simulink model "Loops6"  (Simulink 8.7)
settings: Solver=ode45  StartTime=0.0  StopTime=10.0  RelTol=1e-3
settings Model: Creator=scaife  LastModifiedBy=bourbouh  ExtModeAutoUpdateStatusClock=off
settings DataIOCC: SignalLoggingSaveFormat=ModelDataLogs  SignalLoggingName=sigsOut
settings OptimizationCC: InitFltsAndDblsToZero=on
settings DebuggingCC: SaveWithParameterizedLinksMsg=none  SignalResolutionControl=TryResolveAllWithWarning  MultiTaskDSMMsg=warning  MultiTaskCondExecSysMsg=none
settings HardwareCC: TargetUnknown=on
settings SFSimCC: SimParseCustomCode=off
settings GRTTargetCC: TargetFcnLib=ansi_tfl_tmw.mat  ModelReferenceCompliant=off  GeneratePreprocessorConditionals=Use local settings  CombineOutputUpdateFcns=off  MatFileLogging=off  GRTInterface=on

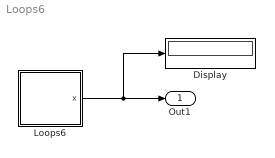
== system Loops6 ==
  Display : Display
  Loops6 : Stateflow chart  TreatAsAtomicUnit=on
  Out1 : Outport
  wires:
  Loops6/1(x) -> Display/1, Out1/1

== stateflow chart Loops6 ==
  state A
  state B
  (default) -> A
  A -> (junction 7) : {x=0;}
  (junction 8) -> (junction 7) [order 1] : [x<4]{x++;}
  (junction 9) -> (junction 7) [order 1] : [x<2]{x++;}
  (junction 7) -> (junction 8) [order 2] : {y=!y;}
  (junction 7) -> (junction 9) [order 1] : [!y]{y=!y;}
  (junction 8) -> B [order 2]
  (junction 9) -> B [order 2]
  data: x output int32; y local boolean
